simulink model "twoFSK"  (R2018a)
settings: Solver=VariableStepAuto  StartTime=0.0  StopTime=40.0  RelTol=1e-3
libraries: dsparch4 x4, commrandsrc3 x1
settings Model: Creator=mengmeng  LastModifiedBy=mengmeng

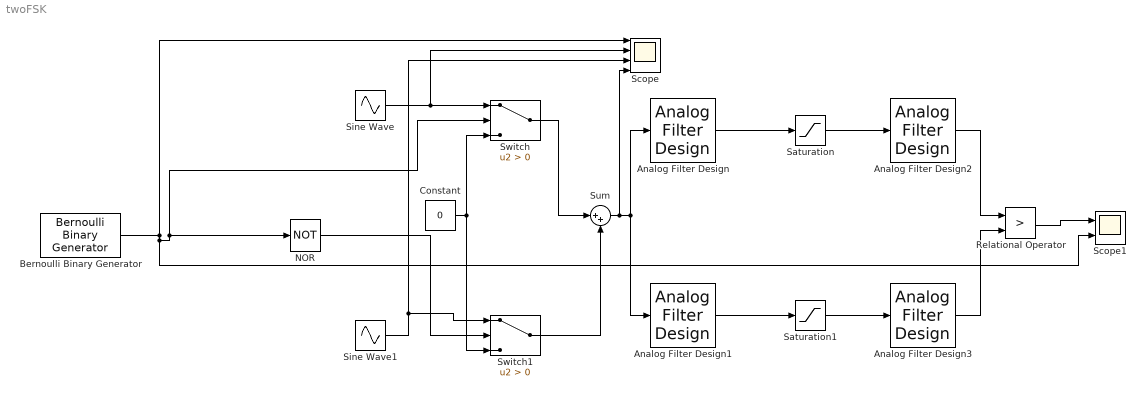
== system twoFSK ==
  Analog Filter Design : dsparch4/Analog Filter Design  method=Butterworth  filttype=Bandpass  N=8  Wlo=80  Whi=120  Rp=2  Rs=40
  Analog Filter Design1 : dsparch4/Analog Filter Design  method=Butterworth  filttype=Bandpass  N=8  Wlo=10  Whi=30  Rp=2  Rs=40
  Analog Filter Design2 : dsparch4/Analog Filter Design  method=Butterworth  filttype=Lowpass  N=8  Wlo=10  Whi=80  Rp=2  Rs=40
  Analog Filter Design3 : dsparch4/Analog Filter Design  method=Butterworth  filttype=Lowpass  N=8  Wlo=30  Whi=80  Rp=2  Rs=40
  Bernoulli Binary Generator : commrandsrc3/Bernoulli Binary Generator  ProbabilityOfZero=0.5  SeedSource=Parameter  Seed=61  SampleTime=1  SamplesPerFrame=1  OutputDataType=uint8  SimulateUsing=Interpreted execution
  Constant : Constant  Value=0
  NOR : Logic  Operator=NOT  Inputs=1  IconShape=distinctive  AllPortsSameDT=off  OutDataTypeStr=uint(8)
  Relational Operator : RelationalOperator  Operator=>  OutDataTypeStr=boolean  RndMeth=Simplest
  Saturation : Saturate  UpperLimit=inf  LowerLimit=0
  Saturation1 : Saturate
  Scope : Scope  NumInputPorts=4
  Scope1 : Scope  NumInputPorts=2
  Sine Wave : Sin  Frequency=100  SampleTime=0
  Sine Wave1 : Sin  Frequency=20  SampleTime=0
  Sum : Sum  Inputs=|++
  Switch : Switch  Criteria=u2 > Threshold
  Switch1 : Switch  Criteria=u2 > Threshold
  wires:
  NOR/1 -> Switch1/2
  Switch1/1 -> Sum/2
  Constant/1 -> Switch/3, Switch1/3
  Sum/1 -> Scope/4, Analog Filter Design1/1, Analog Filter Design/1
  Analog Filter Design/1 -> Saturation/1
  Analog Filter Design1/1 -> Saturation1/1
  Saturation/1 -> Analog Filter Design2/1
  Saturation1/1 -> Analog Filter Design3/1
  Analog Filter Design2/1 -> Relational Operator/1
  Analog Filter Design3/1 -> Relational Operator/2
  Relational Operator/1 -> Scope1/1
  Sine Wave1/1 -> Switch1/1, Scope/3
  Sine Wave/1 -> Switch/1, Scope/2
  Switch/1 -> Sum/1
  Bernoulli Binary Generator/1 -> Scope1/2, NOR/1, Switch/2, Scope/1
